simulink model "unicycle"  (R2017a)
settings: Solver=ode45  StartTime=0.0  StopTime=20  RelTol=1e-3  EnableMultiTasking=on
InitFcn:
  | param
values from neighbouring files (symbols this model uses):
  P = P - Li*C*P    [estimator_ekf.m]    (also in estimator_ukf.m = P - L*S*L'; unscented_transform.m = [1 .5; .5 1])
undefined symbols (not defined in the file or in its folder): draw_unicycle, plot_states, unicycle_sensors
settings Model: Creator=beard  LastModifiedBy=Jacob
settings DataIOCC: LimitDataPoints=on  SaveFormat=Array  SignalLoggingSaveFormat=ModelDataLogs
settings OptimizationCC: ExpressionDepthLimit=2147483647  InitFltsAndDblsToZero=on  LifeSpan=inf
settings DebuggingCC: UnderspecifiedInitializationDetection=Classic  MergeDetectMultiDrivingBlocksExec=none  SolverPrmCheckMsg=warning  FcnCallInpInsideContextMsg=warning  AllowSymbolicDim=off  StateNameClashWarn=warning  SFUnexpectedBacktrackingDiag=warning  SFNoUnconditionalDefaultTransitionDiag=warning  SFExecutionAtInitializationDiag=none
settings HardwareCC: ProdBitPerPointer=32  ProdBitPerSizeT=32  ProdBitPerPtrDiffT=32  ProdLargestAtomicFloat=None  ProdIntDivRoundTo=Undefined  ProdEndianess=Unspecified  ProdWordSize=32  ProdHWDeviceType=32-bit Generic
settings ModelReferenceCC: PropagateSignalLabelsOutOfModel=off
settings GRTTargetCC: TargetLangStandard=C89/C90 (ANSI)  GeneratePreprocessorConditionals=Disable all  CombineOutputUpdateFcns=off  GRTInterface=on
settings ConfigComp: CovMetricSettings=dw  CovHtmlReporting=on  CovSaveCumulativeToWorkspaceVar=on  CovSaveSingleToWorkspaceVar=on  CovExternalEMLEnable=off

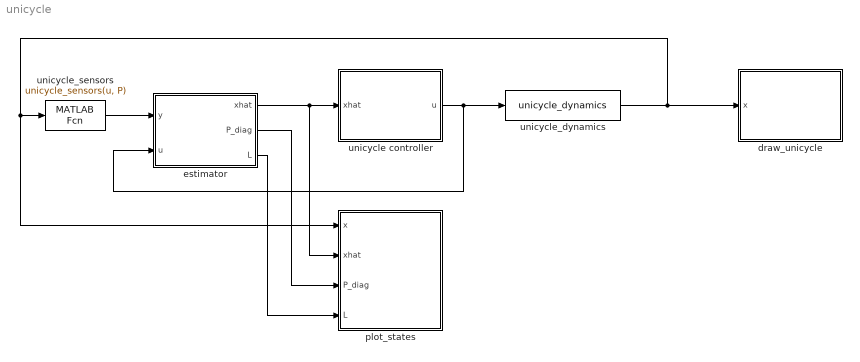
== system unicycle ==
  draw_unicycle : Subsystem
  estimator : Subsystem
  plot_states : Subsystem
  unicycle controller : Subsystem
  unicycle_dynamics : S-Function  FunctionName=unicycle_dynamics  Parameters=P  SFunctionDeploymentMode=off  EnableBusSupport=off
  unicycle_sensors : MATLABFcn  MATLABFcn=unicycle_sensors(u, P)  SampleTime=P.sampleTime
  wires:
  unicycle controller/1(u) -> unicycle_dynamics/1, estimator/2(u)
  unicycle_dynamics/1 -> plot_states/1(x), unicycle_sensors/1, draw_unicycle/1(x)
  unicycle_sensors/1 -> estimator/1(y)
  estimator/1(xhat) -> plot_states/2(xhat), unicycle controller/1(xhat)
  estimator/2(P_diag) -> plot_states/3(P_diag)
  estimator/3(L) -> plot_states/4(L)

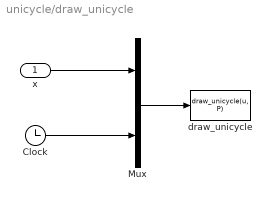
== system unicycle/draw_unicycle ==
  x : Inport
  Clock : Clock
  Mux : Mux  Inputs=2
  draw_unicycle : MATLABFcn  MATLABFcn=draw_unicycle(u, P)  OutputDimensions=0  SampleTime=0.1
  wires:
  x/1 -> Mux/1
  Mux/1 -> draw_unicycle/1
  Clock/1 -> Mux/2

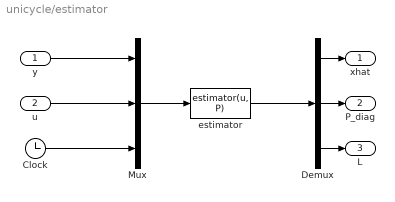
== system unicycle/estimator ==
  y : Inport
  u : Inport  Port=2
  Clock : Clock
  Demux : Demux  Outputs=[3; 3; 1]
  Mux : Mux  Inputs=[size(P.landmarks, 2)*2 2 1]
  estimator : MATLABFcn  MATLABFcn=estimator(u, P)  OutputDimensions=7  SampleTime=P.sampleTime
  xhat : Outport
  P_diag : Outport  Port=2
  L : Outport  Port=3
  wires:
  Clock/1 -> Mux/3
  Mux/1 -> estimator/1
  y/1 -> Mux/1
  u/1 -> Mux/2
  Demux/1 -> xhat/1
  estimator/1 -> Demux/1
  Demux/3 -> L/1
  Demux/2 -> P_diag/1

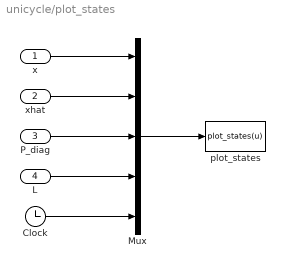
== system unicycle/plot_states ==
  x : Inport
  xhat : Inport  Port=2
  P_diag : Inport  Port=3
  L : Inport  Port=4
  Clock : Clock
  Mux : Mux  Inputs=[3 3 3 1 1]
  plot_states : MATLABFcn  MATLABFcn=plot_states(u)  OutputDimensions=0  SampleTime=P.sampleTime
  wires:
  x/1 -> Mux/1
  Mux/1 -> plot_states/1
  Clock/1 -> Mux/5
  xhat/1 -> Mux/2
  L/1 -> Mux/4
  P_diag/1 -> Mux/3

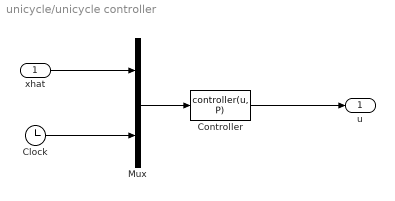
== system unicycle/unicycle controller ==
  xhat : Inport
  Clock : Clock
  Controller : MATLABFcn  MATLABFcn=controller(u, P)  SampleTime=P.sampleTime
  Mux : Mux  Inputs=2
  u : Outport
  wires:
  xhat/1 -> Mux/1
  Mux/1 -> Controller/1
  Clock/1 -> Mux/2
  Controller/1 -> u/1
